simulink library "csu_cmv_convert_measured_voltages_collection_lib"  (R2014b)
settings: Solver=ode45  StartTime=0.0  StopTime=10.0  RelTol=1e-3
libraries: util_info_lib x1
settings Model: Creator=escrane  LastModifiedBy=mstewart

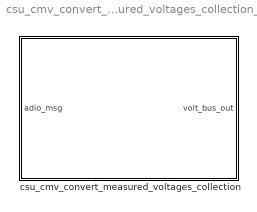
== system csu_cmv_convert_measured_voltages_collection_lib ==
  csu_cmv_convert_measured_voltages_collection : Subsystem
      mask Display: color('blue');text(0.05, 0.02, 'MoonEx', 'HorizontalAlignment', 'Left', 'VerticalAlignment', 'Bottom');color('red');text(0.95, 0.02, 'Autogenerated', 'HorizontalAlignment', 'Right', 'VerticalAlignment', 'Bottom');

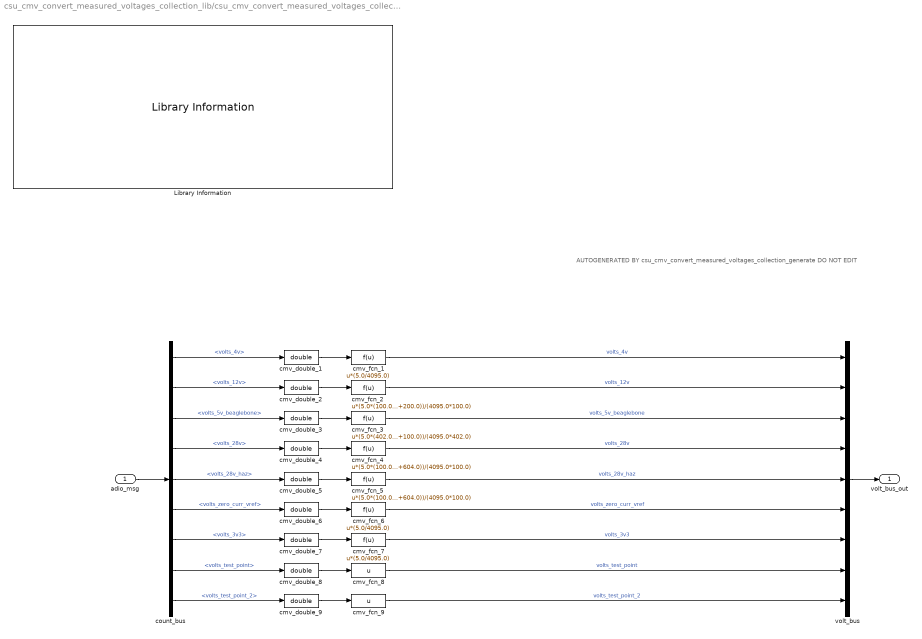
== system csu_cmv_convert_measured_voltages_collection_lib/csu_cmv_convert_measured_voltages_collection ==
  note: AUTOGENERATED BY csu_cmv_convert_measured_voltages_collection_generate
      | DO NOT EDIT
  adio_msg : Inport
  Library Information : util_info_lib/Library Information  owner='escrane'
  cmv_double_{1..9} (9 alike) : DataTypeConversion  OutDataTypeStr=double
  cmv_fcn_1 : Fcn  Expr=u*(5.0/4095.0)
  cmv_fcn_2 : Fcn  Expr=u*(5.0*(100.0+200.0))/(4095.0*100.0)
  cmv_fcn_3 : Fcn  Expr=u*(5.0*(402.0+100.0))/(4095.0*402.0)
  cmv_fcn_4 : Fcn  Expr=u*(5.0*(100.0+604.0))/(4095.0*100.0)
  cmv_fcn_5 : Fcn  Expr=u*(5.0*(100.0+604.0))/(4095.0*100.0)
  cmv_fcn_6 : Fcn  Expr=u*(5.0/4095.0)
  cmv_fcn_7 : Fcn  Expr=u*(5.0/4095.0)
  cmv_fcn_8 : Fcn  Expr=u
  cmv_fcn_9 : Fcn  Expr=u
  count_bus : BusSelector  OutputSignals=volts_4v,volts_12v,volts_5v_beaglebone,volts_28v,volts_28v_haz,volts_zero_curr_vref,volts_3v3,volts_test_point,volts_test_point_2
  volt_bus : BusCreator  Inputs=9
  volt_bus_out : Outport
  wires:
  adio_msg/1 -> count_bus/1
  volt_bus/1 -> volt_bus_out/1
  count_bus/1 -> cmv_double_1/1  "<volts_4v>"
  cmv_double_1/1 -> cmv_fcn_1/1
  cmv_fcn_1/1 -> volt_bus/1  "volts_4v"
  count_bus/2 -> cmv_double_2/1  "<volts_12v>"
  cmv_double_2/1 -> cmv_fcn_2/1
  cmv_fcn_2/1 -> volt_bus/2  "volts_12v"
  count_bus/3 -> cmv_double_3/1  "<volts_5v_beaglebone>"
  cmv_double_3/1 -> cmv_fcn_3/1
  cmv_fcn_3/1 -> volt_bus/3  "volts_5v_beaglebone"
  count_bus/4 -> cmv_double_4/1  "<volts_28v>"
  cmv_double_4/1 -> cmv_fcn_4/1
  cmv_fcn_4/1 -> volt_bus/4  "volts_28v"
  count_bus/5 -> cmv_double_5/1  "<volts_28v_haz>"
  cmv_double_5/1 -> cmv_fcn_5/1
  cmv_fcn_5/1 -> volt_bus/5  "volts_28v_haz"
  count_bus/6 -> cmv_double_6/1  "<volts_zero_curr_vref>"
  cmv_double_6/1 -> cmv_fcn_6/1
  cmv_fcn_6/1 -> volt_bus/6  "volts_zero_curr_vref"
  count_bus/7 -> cmv_double_7/1  "<volts_3v3>"
  cmv_double_7/1 -> cmv_fcn_7/1
  cmv_fcn_7/1 -> volt_bus/7  "volts_3v3"
  count_bus/8 -> cmv_double_8/1  "<volts_test_point>"
  cmv_double_8/1 -> cmv_fcn_8/1
  cmv_fcn_8/1 -> volt_bus/8  "volts_test_point"
  count_bus/9 -> cmv_double_9/1  "<volts_test_point_2>"
  cmv_double_9/1 -> cmv_fcn_9/1
  cmv_fcn_9/1 -> volt_bus/9  "volts_test_point_2"
